simulink model "Test_simulation_model_backhoe"  (R2024a)
settings: Solver=FixedStepAuto  StartTime=0.0  StopTime=inf  FixedStep=0.0001  RelTol=1e-9
undefined symbols (not defined in the file or in its folder): X, Y, Z
libraries: sm_lib x67, nesl_utility x36, slpidlib x8
(part 3 of 4)

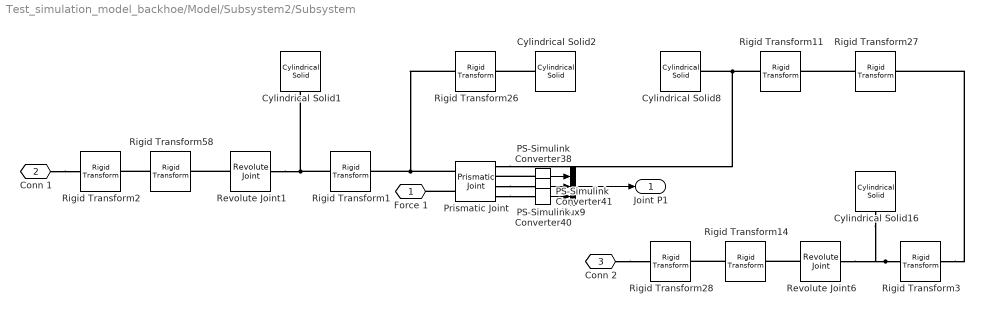
== system Test_simulation_model_backhoe/Model/Subsystem2/Subsystem ==
  Cylindrical Solid1 : sm_lib/Body Elements/Cylindrical Solid  CylinderRadius=0.05  CylinderRadiusUnits=m  CylinderLength=0.1  CylinderLengthUnits=m  ExportEntireGeometry=off  InertiaType=PointMass  BasedOnType=Density  Density=1000  DensityUnits=kg/m^3  Mass=0.0001  MassUnits=kg  CenterOfMass=[0 0 0]  CenterOfMassUnits=m  MomentsOfInertia=[1 1 1]  MomentsOfInertiaUnits=kg*m^2  ProductsOfInertia=[0 0 0]  ProductsOfInertiaUnits=kg*m^2  GraphicType=FromGeometry  MarkerShape=Sphere  MarkerSize=10  GraphicVisPropType=SimpleVisualProperties  GraphicDiffuseColor=[0.8 0.4 1.0]  GraphicOpacity=1.0  GraphicSpecularColor=[0.5 0.5 0.5 1.0]  GraphicAmbientColor=[0.15 0.15 0.15 1.0]  GraphicEmissiveColor=[0.0 0.0 0.0 1.0]  GraphicShininess=75  DoExposeReferenceFrame=on  SerializedFrames=<Frames/>
  Cylindrical Solid16 : sm_lib/Body Elements/Cylindrical Solid  CylinderRadius=0.05  CylinderRadiusUnits=m  CylinderLength=0.1  CylinderLengthUnits=m  ExportEntireGeometry=off  InertiaType=PointMass  BasedOnType=Density  Density=1000  DensityUnits=kg/m^3  Mass=0.00001  MassUnits=kg  CenterOfMass=[0 0 0]  CenterOfMassUnits=m  MomentsOfInertia=[1 1 1]  MomentsOfInertiaUnits=kg*m^2  ProductsOfInertia=[0 0 0]  ProductsOfInertiaUnits=kg*m^2  GraphicType=FromGeometry  MarkerShape=Sphere  MarkerSize=10  GraphicVisPropType=SimpleVisualProperties  GraphicDiffuseColor=[0.8 0.4 1.0]  GraphicOpacity=1.0  GraphicSpecularColor=[0.5 0.5 0.5 1.0]  GraphicAmbientColor=[0.15 0.15 0.15 1.0]  GraphicEmissiveColor=[0.0 0.0 0.0 1.0]  GraphicShininess=75  DoExposeReferenceFrame=on  SerializedFrames=<Frames/>
  Cylindrical Solid2 : sm_lib/Body Elements/Cylindrical Solid  CylinderRadius=0.02  CylinderRadiusUnits=m  CylinderLength=0.4  CylinderLengthUnits=m  ExportEntireGeometry=off  InertiaType=PointMass  BasedOnType=Density  Density=1000  DensityUnits=kg/m^3  Mass=0.001  MassUnits=kg  CenterOfMass=[0 0 0]  CenterOfMassUnits=m  MomentsOfInertia=[1 1 1]  MomentsOfInertiaUnits=kg*m^2  ProductsOfInertia=[0 0 0]  ProductsOfInertiaUnits=kg*m^2  GraphicType=FromGeometry  MarkerShape=Sphere  MarkerSize=10  GraphicVisPropType=SimpleVisualProperties  GraphicDiffuseColor=[0.0 0.8 0.6]  GraphicOpacity=1.0  GraphicSpecularColor=[0.5 0.5 0.5 1.0]  GraphicAmbientColor=[0.15 0.15 0.15 1.0]  GraphicEmissiveColor=[0.0 0.0 0.0 1.0]  GraphicShininess=75  DoExposeReferenceFrame=on  SerializedFrames=<Frames/>
  Cylindrical Solid8 : sm_lib/Body Elements/Cylindrical Solid  CylinderRadius=0.01  CylinderRadiusUnits=m  CylinderLength=0.55  CylinderLengthUnits=m  ExportEntireGeometry=off  InertiaType=PointMass  BasedOnType=Density  Density=1000  DensityUnits=kg/m^3  Mass=0.001  MassUnits=kg  CenterOfMass=[0 0 0]  CenterOfMassUnits=m  MomentsOfInertia=[1 1 1]  MomentsOfInertiaUnits=kg*m^2  ProductsOfInertia=[0 0 0]  ProductsOfInertiaUnits=kg*m^2  GraphicType=FromGeometry  MarkerShape=Sphere  MarkerSize=10  GraphicVisPropType=SimpleVisualProperties  GraphicDiffuseColor=[0.2 0.8 1.0]  GraphicOpacity=1.0  GraphicSpecularColor=[0.5 0.5 0.5 1.0]  GraphicAmbientColor=[0.15 0.15 0.15 1.0]  GraphicEmissiveColor=[0.0 0.0 0.0 1.0]  GraphicShininess=75  DoExposeReferenceFrame=on  SerializedFrames=<Frames/>
  Mux9 : Mux  Inputs=3
  PS-Simulink Converter38 : nesl_utility/PS-Simulink Converter  PhysicalDomain=network_engine_domain  SubClassName=ps_output  LeftPortType=input  RightPortType=output  PseudoPeriodic=off  Frequencies=[]  VectorFormat=inherit  Unit=inherit  AffineConversion=off
  PS-Simulink Converter40 : nesl_utility/PS-Simulink Converter  PhysicalDomain=network_engine_domain  SubClassName=ps_output  LeftPortType=input  RightPortType=output  PseudoPeriodic=off  Frequencies=[]  VectorFormat=inherit  Unit=inherit  AffineConversion=off
  PS-Simulink Converter41 : nesl_utility/PS-Simulink Converter  PhysicalDomain=network_engine_domain  SubClassName=ps_output  LeftPortType=input  RightPortType=output  PseudoPeriodic=off  Frequencies=[]  VectorFormat=inherit  Unit=inherit  AffineConversion=off
  Prismatic Joint : sm_lib/Joints/Prismatic Joint  JointMode=Normal  CompositeWrenchDir=FollowerOnBase  CompositeWrenchFrame=BaseFrame  SenseConstraintForce=off  SenseConstraintTorque=off  SenseTotalForce=off  SenseTotalTorque=off  PositionTargetSpecify=off  PositionTargetPriority=High  PositionTargetValue=0  PositionTargetValueUnits=m  VelocityTargetSpecify=off  VelocityTargetPriority=High  VelocityTargetValue=0  VelocityTargetValueUnits=m/s  EquilibriumPosition=0  EquilibriumPositionUnits=m  SpringStiffness=0  SpringStiffnessUnits=N/m  DampingCoefficient=0  DampingCoefficientUnits=N/(m/s)  LowerLimitSpecify=on  LowerLimitBound=0.25  LowerLimitBoundUnits=m  LowerLimitStiffness=1e6  LowerLimitStiffnessUnits=N/m  LowerLimitDamping=1e3  LowerLimitDampingUnits=N/(m/s)  LowerLimitTransitionRegionWidth=1e-4  LowerLimitTransitionRegionWidthUnits=m  UpperLimitSpecify=on  UpperLimitBound=0.6  UpperLimitBoundUnits=m  UpperLimitStiffness=1e6  UpperLimitStiffnessUnits=N/m  UpperLimitDamping=1e3  UpperLimitDampingUnits=N/(m/s)  UpperLimitTransitionRegionWidth=1e-4  UpperLimitTransitionRegionWidthUnits=m  TorqueActuationMode=InputTorque  MotionActuationMode=ComputedMotion  SensePosition=on  SenseVelocity=on  SenseAcceleration=off  SenseTorqueForce=on  SenseLowerLimitTorqueForce=off  SenseUpperLimitTorqueForce=off
  Revolute Joint1 : sm_lib/Joints/Revolute Joint  JointMode=Normal  CompositeWrenchDir=FollowerOnBase  CompositeWrenchFrame=BaseFrame  SenseConstraintForce=off  SenseConstraintTorque=off  SenseTotalForce=off  SenseTotalTorque=off  PositionTargetSpecify=on  PositionTargetPriority=Low  PositionTargetValue=-60  PositionTargetValueUnits=deg  VelocityTargetSpecify=off  VelocityTargetPriority=High  VelocityTargetValue=0  VelocityTargetValueUnits=deg/s  EquilibriumPosition=0  EquilibriumPositionUnits=deg  SpringStiffness=0  SpringStiffnessUnits=N*m/deg  DampingCoefficient=0  DampingCoefficientUnits=N*m/(deg/s)  LowerLimitSpecify=off  LowerLimitBound=-2  LowerLimitBoundUnits=deg  LowerLimitStiffness=1e4  LowerLimitStiffnessUnits=N*m/deg  LowerLimitDamping=10  LowerLimitDampingUnits=N*m/(deg/s)  LowerLimitTransitionRegionWidth=0.1  LowerLimitTransitionRegionWidthUnits=deg  UpperLimitSpecify=off  UpperLimitBound=-1  UpperLimitBoundUnits=deg  UpperLimitStiffness=1e4  UpperLimitStiffnessUnits=N*m/deg  UpperLimitDamping=10  UpperLimitDampingUnits=N*m/(deg/s)  UpperLimitTransitionRegionWidth=0.1  UpperLimitTransitionRegionWidthUnits=deg  TorqueActuationMode=NoTorque  MotionActuationMode=ComputedMotion  SensePosition=off  SenseVelocity=off  SenseAcceleration=off  SenseTorqueForce=off  SenseLowerLimitTorqueForce=off  SenseUpperLimitTorqueForce=off
  Revolute Joint6 : sm_lib/Joints/Revolute Joint  JointMode=Normal  CompositeWrenchDir=FollowerOnBase  CompositeWrenchFrame=BaseFrame  SenseConstraintForce=off  SenseConstraintTorque=off  SenseTotalForce=off  SenseTotalTorque=off  PositionTargetSpecify=off  PositionTargetPriority=High  PositionTargetValue=0  PositionTargetValueUnits=deg  VelocityTargetSpecify=off  VelocityTargetPriority=High  VelocityTargetValue=0  VelocityTargetValueUnits=deg/s  EquilibriumPosition=0  EquilibriumPositionUnits=deg  SpringStiffness=0  SpringStiffnessUnits=N*m/deg  DampingCoefficient=0  DampingCoefficientUnits=N*m/(deg/s)  LowerLimitSpecify=off  LowerLimitBound=-90  LowerLimitBoundUnits=deg  LowerLimitStiffness=1e4  LowerLimitStiffnessUnits=N*m/deg  LowerLimitDamping=10  LowerLimitDampingUnits=N*m/(deg/s)  LowerLimitTransitionRegionWidth=0.1  LowerLimitTransitionRegionWidthUnits=deg  UpperLimitSpecify=off  UpperLimitBound=90  UpperLimitBoundUnits=deg  UpperLimitStiffness=1e4  UpperLimitStiffnessUnits=N*m/deg  UpperLimitDamping=10  UpperLimitDampingUnits=N*m/(deg/s)  UpperLimitTransitionRegionWidth=0.1  UpperLimitTransitionRegionWidthUnits=deg  TorqueActuationMode=NoTorque  MotionActuationMode=ComputedMotion  SensePosition=off  SenseVelocity=off  SenseAcceleration=off  SenseTorqueForce=off  SenseLowerLimitTorqueForce=off  SenseUpperLimitTorqueForce=off
  Rigid Transform1 : sm_lib/Frames and Transforms/Rigid Transform  RotationMethod=StandardAxis  FollAlignAxisA=+X  BaseAlignAxisA=+Y  FollAlignAxisB=+Y  BaseAlignAxisB=+Z  RotationStandardAxis=-X  RotationAngle=90  RotationAngleUnits=deg  RotationArbitraryAxis=[0 0 1]  RotationSequenceAxes=FollowerAxes  RotationSequence=XYX  RotationSequenceAngles=[0 0 0]  RotationSequenceAnglesUnits=deg  RotationMatrix=[1 0 0; 0 1 0; 0 0 1]  Quaternion=[1 0 0 0]  TranslationMethod=Cartesian  TranslationCartesianOffset=[0 0 0]  TranslationCartesianOffsetUnits=m  TranslationStandardAxis=+Z  TranslationStandardOffset=0  TranslationStandardOffsetUnits=m  TranslationROffset=0  TranslationROffsetUnits=m  TranslationThetaOffset=0  TranslationThetaOffsetUnits=deg  TranslationZOffset=0  TranslationZOffsetUnits=m
  Rigid Transform11 : sm_lib/Frames and Transforms/Rigid Transform  RotationMethod=StandardAxis  FollAlignAxisA=+X  BaseAlignAxisA=+Y  FollAlignAxisB=+Y  BaseAlignAxisB=+Z  RotationStandardAxis=-Z  RotationAngle=90  RotationAngleUnits=deg  RotationArbitraryAxis=[0 0 1]  RotationSequenceAxes=FollowerAxes  RotationSequence=XYX  RotationSequenceAngles=[0 0 0]  RotationSequenceAnglesUnits=deg  RotationMatrix=[1 0 0; 0 1 0; 0 0 1]  Quaternion=[1 0 0 0]  TranslationMethod=Cartesian  TranslationCartesianOffset=[0 0 0]  TranslationCartesianOffsetUnits=m  TranslationStandardAxis=+Z  TranslationStandardOffset=0  TranslationStandardOffsetUnits=m  TranslationROffset=0  TranslationROffsetUnits=m  TranslationThetaOffset=0  TranslationThetaOffsetUnits=deg  TranslationZOffset=0  TranslationZOffsetUnits=m
  Rigid Transform14 : sm_lib/Frames and Transforms/Rigid Transform  RotationMethod=StandardAxis  FollAlignAxisA=+X  BaseAlignAxisA=+Y  FollAlignAxisB=+Y  BaseAlignAxisB=+Z  RotationStandardAxis=-Y  RotationAngle=90  RotationAngleUnits=deg  RotationArbitraryAxis=[0 0 1]  RotationSequenceAxes=FollowerAxes  RotationSequence=XYX  RotationSequenceAngles=[0 0 0]  RotationSequenceAnglesUnits=deg  RotationMatrix=[1 0 0; 0 1 0; 0 0 1]  Quaternion=[1 0 0 0]  TranslationMethod=Cartesian  TranslationCartesianOffset=[0 0 0]  TranslationCartesianOffsetUnits=m  TranslationStandardAxis=+Z  TranslationStandardOffset=0  TranslationStandardOffsetUnits=m  TranslationROffset=0  TranslationROffsetUnits=m  TranslationThetaOffset=0  TranslationThetaOffsetUnits=deg  TranslationZOffset=0  TranslationZOffsetUnits=m
  Rigid Transform2 : sm_lib/Frames and Transforms/Rigid Transform  RotationMethod=StandardAxis  FollAlignAxisA=+X  BaseAlignAxisA=+Y  FollAlignAxisB=+Y  BaseAlignAxisB=+Z  RotationStandardAxis=-Y  RotationAngle=90  RotationAngleUnits=deg  RotationArbitraryAxis=[0 0 1]  RotationSequenceAxes=FollowerAxes  RotationSequence=XYX  RotationSequenceAngles=[0 0 0]  RotationSequenceAnglesUnits=deg  RotationMatrix=[1 0 0; 0 1 0; 0 0 1]  Quaternion=[1 0 0 0]  TranslationMethod=Cartesian  TranslationCartesianOffset=[0 0 0]  TranslationCartesianOffsetUnits=m  TranslationStandardAxis=+Z  TranslationStandardOffset=0  TranslationStandardOffsetUnits=m  TranslationROffset=0  TranslationROffsetUnits=m  TranslationThetaOffset=0  TranslationThetaOffsetUnits=deg  TranslationZOffset=0  TranslationZOffsetUnits=m
  Rigid Transform26 : sm_lib/Frames and Transforms/Rigid Transform  RotationMethod=None  FollAlignAxisA=+X  BaseAlignAxisA=+Y  FollAlignAxisB=+Y  BaseAlignAxisB=+Z  RotationStandardAxis=+Y  RotationAngle=90  RotationAngleUnits=deg  RotationArbitraryAxis=[0 0 1]  RotationSequenceAxes=FollowerAxes  RotationSequence=XYX  RotationSequenceAngles=[0 0 0]  RotationSequenceAnglesUnits=deg  RotationMatrix=[1 0 0; 0 1 0; 0 0 1]  Quaternion=[1 0 0 0]  TranslationMethod=Cartesian  TranslationCartesianOffset=[0 0 0.2]  TranslationCartesianOffsetUnits=m  TranslationStandardAxis=+Z  TranslationStandardOffset=0  TranslationStandardOffsetUnits=m  TranslationROffset=0  TranslationROffsetUnits=m  TranslationThetaOffset=0  TranslationThetaOffsetUnits=deg  TranslationZOffset=0  TranslationZOffsetUnits=m
  Rigid Transform27 : sm_lib/Frames and Transforms/Rigid Transform  RotationMethod=None  FollAlignAxisA=+X  BaseAlignAxisA=+Y  FollAlignAxisB=+Y  BaseAlignAxisB=+Z  RotationStandardAxis=+Y  RotationAngle=90  RotationAngleUnits=deg  RotationArbitraryAxis=[0 0 1]  RotationSequenceAxes=FollowerAxes  RotationSequence=XYX  RotationSequenceAngles=[0 0 0]  RotationSequenceAnglesUnits=deg  RotationMatrix=[1 0 0; 0 1 0; 0 0 1]  Quaternion=[1 0 0 0]  TranslationMethod=Cartesian  TranslationCartesianOffset=[0 0 -0.3]  TranslationCartesianOffsetUnits=m  TranslationStandardAxis=+Z  TranslationStandardOffset=0  TranslationStandardOffsetUnits=m  TranslationROffset=0  TranslationROffsetUnits=m  TranslationThetaOffset=0  TranslationThetaOffsetUnits=deg  TranslationZOffset=0  TranslationZOffsetUnits=m
  Rigid Transform28 : sm_lib/Frames and Transforms/Rigid Transform  RotationMethod=None  FollAlignAxisA=+X  BaseAlignAxisA=+Y  FollAlignAxisB=+Y  BaseAlignAxisB=+Z  RotationStandardAxis=+Y  RotationAngle=90  RotationAngleUnits=deg  RotationArbitraryAxis=[0 0 1]  RotationSequenceAxes=FollowerAxes  RotationSequence=XYX  RotationSequenceAngles=[0 0 0]  RotationSequenceAnglesUnits=deg  RotationMatrix=[1 0 0; 0 1 0; 0 0 1]  Quaternion=[1 0 0 0]  TranslationMethod=Cartesian  TranslationCartesianOffset=[0 0 0.5]  TranslationCartesianOffsetUnits=m  TranslationStandardAxis=+Z  TranslationStandardOffset=0  TranslationStandardOffsetUnits=m  TranslationROffset=0  TranslationROffsetUnits=m  TranslationThetaOffset=0  TranslationThetaOffsetUnits=deg  TranslationZOffset=0  TranslationZOffsetUnits=m
  Rigid Transform3 : sm_lib/Frames and Transforms/Rigid Transform  RotationMethod=StandardAxis  FollAlignAxisA=+X  BaseAlignAxisA=+Y  FollAlignAxisB=+Y  BaseAlignAxisB=+Z  RotationStandardAxis=+Y  RotationAngle=90  RotationAngleUnits=deg  RotationArbitraryAxis=[0 0 1]  RotationSequenceAxes=FollowerAxes  RotationSequence=XYX  RotationSequenceAngles=[0 0 0]  RotationSequenceAnglesUnits=deg  RotationMatrix=[1 0 0; 0 1 0; 0 0 1]  Quaternion=[1 0 0 0]  TranslationMethod=Cartesian  TranslationCartesianOffset=[0 0 0]  TranslationCartesianOffsetUnits=m  TranslationStandardAxis=+Z  TranslationStandardOffset=0  TranslationStandardOffsetUnits=m  TranslationROffset=0  TranslationROffsetUnits=m  TranslationThetaOffset=0  TranslationThetaOffsetUnits=deg  TranslationZOffset=0  TranslationZOffsetUnits=m
  Rigid Transform58 : sm_lib/Frames and Transforms/Rigid Transform  RotationMethod=None  FollAlignAxisA=+X  BaseAlignAxisA=+Y  FollAlignAxisB=+Y  BaseAlignAxisB=+Z  RotationStandardAxis=-Y  RotationAngle=90  RotationAngleUnits=deg  RotationArbitraryAxis=[0 0 1]  RotationSequenceAxes=FollowerAxes  RotationSequence=XYX  RotationSequenceAngles=[0 0 0]  RotationSequenceAnglesUnits=deg  RotationMatrix=[1 0 0; 0 1 0; 0 0 1]  Quaternion=[1 0 0 0]  TranslationMethod=Cartesian  TranslationCartesianOffset=[0 0 0]  TranslationCartesianOffsetUnits=m  TranslationStandardAxis=+Z  TranslationStandardOffset=0  TranslationStandardOffsetUnits=m  TranslationROffset=0  TranslationROffsetUnits=m  TranslationThetaOffset=0  TranslationThetaOffsetUnits=deg  TranslationZOffset=0  TranslationZOffsetUnits=m
  Force 1 : PMIOPort  Side=Left
  Conn 1 : PMIOPort  Port=2  Side=Left
  Conn 2 : PMIOPort  Port=3  Side=Left
  Joint P1 : Outport
  wires:
  PS-Simulink Converter40/1 -> Mux9/2
  PS-Simulink Converter38/1 -> Mux9/1
  Mux9/1 -> Joint P1/1
  PS-Simulink Converter41/1 -> Mux9/3
  connections:
  Rigid Transform26/LConn1 -- Prismatic Joint/LConn1 -- Rigid Transform1/RConn1
  Rigid Transform27/RConn1 -- Rigid Transform11/LConn1
  PS-Simulink Converter38/LConn1 -- Prismatic Joint/RConn2
  Rigid Transform11/RConn1 -- Prismatic Joint/RConn1 -- Cylindrical Solid8/RConn1
  Rigid Transform58/LConn1 -- Rigid Transform2/RConn1
  Revolute Joint6/LConn1 -- Rigid Transform14/RConn1
  Rigid Transform3/RConn1 -- Rigid Transform27/LConn1
  Rigid Transform3/LConn1 -- Cylindrical Solid16/RConn1 -- Revolute Joint6/RConn1
  Cylindrical Solid2/RConn1 -- Rigid Transform26/RConn1
  Rigid Transform14/LConn1 -- Rigid Transform28/RConn1
  Conn 2/RConn1 -- Rigid Transform28/LConn1
  Rigid Transform1/LConn1 -- Revolute Joint1/RConn1 -- Cylindrical Solid1/RConn1
  Conn 1/RConn1 -- Rigid Transform2/LConn1
  Revolute Joint1/LConn1 -- Rigid Transform58/RConn1
  Prismatic Joint/RConn4 -- PS-Simulink Converter41/LConn1
  Prismatic Joint/RConn3 -- PS-Simulink Converter40/LConn1
  Prismatic Joint/LConn2 -- Force 1/RConn1

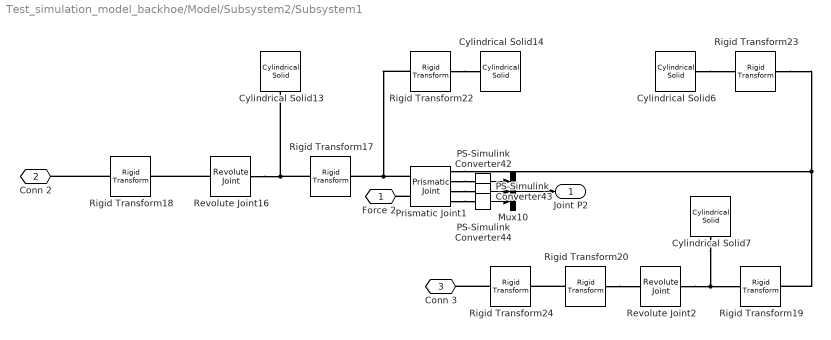
== system Test_simulation_model_backhoe/Model/Subsystem2/Subsystem1 ==
  Cylindrical Solid13 : sm_lib/Body Elements/Cylindrical Solid  CylinderRadius=0.05  CylinderRadiusUnits=m  CylinderLength=0.1  CylinderLengthUnits=m  ExportEntireGeometry=off  InertiaType=PointMass  BasedOnType=Density  Density=1000  DensityUnits=kg/m^3  Mass=0.00001  MassUnits=kg  CenterOfMass=[0 0 0]  CenterOfMassUnits=m  MomentsOfInertia=[1 1 1]  MomentsOfInertiaUnits=kg*m^2  ProductsOfInertia=[0 0 0]  ProductsOfInertiaUnits=kg*m^2  GraphicType=FromGeometry  MarkerShape=Sphere  MarkerSize=10  GraphicVisPropType=SimpleVisualProperties  GraphicDiffuseColor=[0.8 0.4 1.0]  GraphicOpacity=1.0  GraphicSpecularColor=[0.5 0.5 0.5 1.0]  GraphicAmbientColor=[0.15 0.15 0.15 1.0]  GraphicEmissiveColor=[0.0 0.0 0.0 1.0]  GraphicShininess=75  DoExposeReferenceFrame=on  SerializedFrames=<Frames/>
  Cylindrical Solid14 : sm_lib/Body Elements/Cylindrical Solid  CylinderRadius=0.02  CylinderRadiusUnits=m  CylinderLength=0.3  CylinderLengthUnits=m  ExportEntireGeometry=off  InertiaType=PointMass  BasedOnType=Density  Density=1000  DensityUnits=kg/m^3  Mass=0.001  MassUnits=kg  CenterOfMass=[0 0 0]  CenterOfMassUnits=m  MomentsOfInertia=[1 1 1]  MomentsOfInertiaUnits=kg*m^2  ProductsOfInertia=[0 0 0]  ProductsOfInertiaUnits=kg*m^2  GraphicType=FromGeometry  MarkerShape=Sphere  MarkerSize=10  GraphicVisPropType=SimpleVisualProperties  GraphicDiffuseColor=[0.0 0.8 0.6]  GraphicOpacity=1.0  GraphicSpecularColor=[0.5 0.5 0.5 1.0]  GraphicAmbientColor=[0.15 0.15 0.15 1.0]  GraphicEmissiveColor=[0.0 0.0 0.0 1.0]  GraphicShininess=75  DoExposeReferenceFrame=on  SerializedFrames=<Frames/>
  Cylindrical Solid6 : sm_lib/Body Elements/Cylindrical Solid  CylinderRadius=0.01  CylinderRadiusUnits=m  CylinderLength=0.5  CylinderLengthUnits=m  ExportEntireGeometry=off  InertiaType=PointMass  BasedOnType=Density  Density=1000  DensityUnits=kg/m^3  Mass=0.001  MassUnits=kg  CenterOfMass=[0 0 0]  CenterOfMassUnits=m  MomentsOfInertia=[1 1 1]  MomentsOfInertiaUnits=kg*m^2  ProductsOfInertia=[0 0 0]  ProductsOfInertiaUnits=kg*m^2  GraphicType=FromGeometry  MarkerShape=Sphere  MarkerSize=10  GraphicVisPropType=SimpleVisualProperties  GraphicDiffuseColor=[0.2 0.8 1.0]  GraphicOpacity=1.0  GraphicSpecularColor=[0.5 0.5 0.5 1.0]  GraphicAmbientColor=[0.15 0.15 0.15 1.0]  GraphicEmissiveColor=[0.0 0.0 0.0 1.0]  GraphicShininess=75  DoExposeReferenceFrame=on  SerializedFrames=<Frames/>
  Cylindrical Solid7 : sm_lib/Body Elements/Cylindrical Solid  CylinderRadius=0.05  CylinderRadiusUnits=m  CylinderLength=0.1  CylinderLengthUnits=m  ExportEntireGeometry=off  InertiaType=PointMass  BasedOnType=Density  Density=1000  DensityUnits=kg/m^3  Mass=0.00001  MassUnits=kg  CenterOfMass=[0 0 0]  CenterOfMassUnits=m  MomentsOfInertia=[1 1 1]  MomentsOfInertiaUnits=kg*m^2  ProductsOfInertia=[0 0 0]  ProductsOfInertiaUnits=kg*m^2  GraphicType=FromGeometry  MarkerShape=Sphere  MarkerSize=10  GraphicVisPropType=SimpleVisualProperties  GraphicDiffuseColor=[0.8 0.4 1.0]  GraphicOpacity=1.0  GraphicSpecularColor=[0.5 0.5 0.5 1.0]  GraphicAmbientColor=[0.15 0.15 0.15 1.0]  GraphicEmissiveColor=[0.0 0.0 0.0 1.0]  GraphicShininess=75  DoExposeReferenceFrame=on  SerializedFrames=<Frames/>
  Mux10 : Mux  Inputs=3
  PS-Simulink Converter42 : nesl_utility/PS-Simulink Converter  PhysicalDomain=network_engine_domain  SubClassName=ps_output  LeftPortType=input  RightPortType=output  PseudoPeriodic=off  Frequencies=[]  VectorFormat=inherit  Unit=inherit  AffineConversion=off
  PS-Simulink Converter43 : nesl_utility/PS-Simulink Converter  PhysicalDomain=network_engine_domain  SubClassName=ps_output  LeftPortType=input  RightPortType=output  PseudoPeriodic=off  Frequencies=[]  VectorFormat=inherit  Unit=inherit  AffineConversion=off
  PS-Simulink Converter44 : nesl_utility/PS-Simulink Converter  PhysicalDomain=network_engine_domain  SubClassName=ps_output  LeftPortType=input  RightPortType=output  PseudoPeriodic=off  Frequencies=[]  VectorFormat=inherit  Unit=inherit  AffineConversion=off
  Prismatic Joint1 : sm_lib/Joints/Prismatic Joint  JointMode=Normal  CompositeWrenchDir=FollowerOnBase  CompositeWrenchFrame=BaseFrame  SenseConstraintForce=off  SenseConstraintTorque=off  SenseTotalForce=off  SenseTotalTorque=off  PositionTargetSpecify=off  PositionTargetPriority=High  PositionTargetValue=0  PositionTargetValueUnits=m  VelocityTargetSpecify=off  VelocityTargetPriority=High  VelocityTargetValue=0  VelocityTargetValueUnits=m/s  EquilibriumPosition=0  EquilibriumPositionUnits=m  SpringStiffness=0  SpringStiffnessUnits=N/m  DampingCoefficient=0  DampingCoefficientUnits=N/(m/s)  LowerLimitSpecify=on  LowerLimitBound=-0.8  LowerLimitBoundUnits=m  LowerLimitStiffness=1e6  LowerLimitStiffnessUnits=N/m  LowerLimitDamping=1e3  LowerLimitDampingUnits=N/(m/s)  LowerLimitTransitionRegionWidth=1e-4  LowerLimitTransitionRegionWidthUnits=m  UpperLimitSpecify=on  UpperLimitBound=-0.4  UpperLimitBoundUnits=m  UpperLimitStiffness=1e6  UpperLimitStiffnessUnits=N/m  UpperLimitDamping=1e3  UpperLimitDampingUnits=N/(m/s)  UpperLimitTransitionRegionWidth=1e-4  UpperLimitTransitionRegionWidthUnits=m  TorqueActuationMode=InputTorque  MotionActuationMode=ComputedMotion  SensePosition=on  SenseVelocity=on  SenseAcceleration=off  SenseTorqueForce=on  SenseLowerLimitTorqueForce=off  SenseUpperLimitTorqueForce=off
  Revolute Joint16 : sm_lib/Joints/Revolute Joint  JointMode=Normal  CompositeWrenchDir=FollowerOnBase  CompositeWrenchFrame=BaseFrame  SenseConstraintForce=off  SenseConstraintTorque=off  SenseTotalForce=off  SenseTotalTorque=off  PositionTargetSpecify=on  PositionTargetPriority=High  PositionTargetValue=10  PositionTargetValueUnits=deg  VelocityTargetSpecify=off  VelocityTargetPriority=High  VelocityTargetValue=0  VelocityTargetValueUnits=deg/s  EquilibriumPosition=0  EquilibriumPositionUnits=deg  SpringStiffness=0  SpringStiffnessUnits=N*m/deg  DampingCoefficient=0  DampingCoefficientUnits=N*m/(deg/s)  LowerLimitSpecify=off  LowerLimitBound=-45  LowerLimitBoundUnits=deg  LowerLimitStiffness=1e4  LowerLimitStiffnessUnits=N*m/deg  LowerLimitDamping=10  LowerLimitDampingUnits=N*m/(deg/s)  LowerLimitTransitionRegionWidth=0.1  LowerLimitTransitionRegionWidthUnits=deg  UpperLimitSpecify=off  UpperLimitBound=60  UpperLimitBoundUnits=deg  UpperLimitStiffness=1e4  UpperLimitStiffnessUnits=N*m/deg  UpperLimitDamping=10  UpperLimitDampingUnits=N*m/(deg/s)  UpperLimitTransitionRegionWidth=0.1  UpperLimitTransitionRegionWidthUnits=deg  TorqueActuationMode=NoTorque  MotionActuationMode=ComputedMotion  SensePosition=off  SenseVelocity=off  SenseAcceleration=off  SenseTorqueForce=off  SenseLowerLimitTorqueForce=off  SenseUpperLimitTorqueForce=off
  Revolute Joint2 : sm_lib/Joints/Revolute Joint  JointMode=Normal  CompositeWrenchDir=FollowerOnBase  CompositeWrenchFrame=BaseFrame  SenseConstraintForce=off  SenseConstraintTorque=off  SenseTotalForce=off  SenseTotalTorque=off  PositionTargetSpecify=off  PositionTargetPriority=High  PositionTargetValue=0  PositionTargetValueUnits=deg  VelocityTargetSpecify=off  VelocityTargetPriority=High  VelocityTargetValue=0  VelocityTargetValueUnits=deg/s  EquilibriumPosition=0  EquilibriumPositionUnits=deg  SpringStiffness=0  SpringStiffnessUnits=N*m/deg  DampingCoefficient=0  DampingCoefficientUnits=N*m/(deg/s)  LowerLimitSpecify=off  LowerLimitBound=-90  LowerLimitBoundUnits=deg  LowerLimitStiffness=1e4  LowerLimitStiffnessUnits=N*m/deg  LowerLimitDamping=10  LowerLimitDampingUnits=N*m/(deg/s)  LowerLimitTransitionRegionWidth=0.1  LowerLimitTransitionRegionWidthUnits=deg  UpperLimitSpecify=off  UpperLimitBound=90  UpperLimitBoundUnits=deg  UpperLimitStiffness=1e4  UpperLimitStiffnessUnits=N*m/deg  UpperLimitDamping=10  UpperLimitDampingUnits=N*m/(deg/s)  UpperLimitTransitionRegionWidth=0.1  UpperLimitTransitionRegionWidthUnits=deg  TorqueActuationMode=NoTorque  MotionActuationMode=ComputedMotion  SensePosition=off  SenseVelocity=off  SenseAcceleration=off  SenseTorqueForce=off  SenseLowerLimitTorqueForce=off  SenseUpperLimitTorqueForce=off
  Rigid Transform17 : sm_lib/Frames and Transforms/Rigid Transform  RotationMethod=StandardAxis  FollAlignAxisA=+X  BaseAlignAxisA=+Y  FollAlignAxisB=+Y  BaseAlignAxisB=+Z  RotationStandardAxis=-X  RotationAngle=90  RotationAngleUnits=deg  RotationArbitraryAxis=[0 0 1]  RotationSequenceAxes=FollowerAxes  RotationSequence=XYX  RotationSequenceAngles=[0 0 0]  RotationSequenceAnglesUnits=deg  RotationMatrix=[1 0 0; 0 1 0; 0 0 1]  Quaternion=[1 0 0 0]  TranslationMethod=Cartesian  TranslationCartesianOffset=[0 0 0]  TranslationCartesianOffsetUnits=m  TranslationStandardAxis=+Z  TranslationStandardOffset=0  TranslationStandardOffsetUnits=m  TranslationROffset=0  TranslationROffsetUnits=m  TranslationThetaOffset=0  TranslationThetaOffsetUnits=deg  TranslationZOffset=0  TranslationZOffsetUnits=m
  Rigid Transform18 : sm_lib/Frames and Transforms/Rigid Transform  RotationMethod=StandardAxis  FollAlignAxisA=+X  BaseAlignAxisA=+Y  FollAlignAxisB=+Y  BaseAlignAxisB=+Z  RotationStandardAxis=-Y  RotationAngle=90  RotationAngleUnits=deg  RotationArbitraryAxis=[0 0 1]  RotationSequenceAxes=FollowerAxes  RotationSequence=XYX  RotationSequenceAngles=[0 0 0]  RotationSequenceAnglesUnits=deg  RotationMatrix=[1 0 0; 0 1 0; 0 0 1]  Quaternion=[1 0 0 0]  TranslationMethod=Cartesian  TranslationCartesianOffset=[0 0 0.85]  TranslationCartesianOffsetUnits=m  TranslationStandardAxis=+Z  TranslationStandardOffset=0  TranslationStandardOffsetUnits=m  TranslationROffset=0  TranslationROffsetUnits=m  TranslationThetaOffset=0  TranslationThetaOffsetUnits=deg  TranslationZOffset=0  TranslationZOffsetUnits=m
  Rigid Transform19 : sm_lib/Frames and Transforms/Rigid Transform  RotationMethod=StandardAxis  FollAlignAxisA=+X  BaseAlignAxisA=+Y  FollAlignAxisB=+Y  BaseAlignAxisB=+Z  RotationStandardAxis=+X  RotationAngle=90  RotationAngleUnits=deg  RotationArbitraryAxis=[0 0 1]  RotationSequenceAxes=FollowerAxes  RotationSequence=XYX  RotationSequenceAngles=[0 0 0]  RotationSequenceAnglesUnits=deg  RotationMatrix=[1 0 0; 0 1 0; 0 0 1]  Quaternion=[1 0 0 0]  TranslationMethod=Cartesian  TranslationCartesianOffset=[0 0 0]  TranslationCartesianOffsetUnits=m  TranslationStandardAxis=+Z  TranslationStandardOffset=0  TranslationStandardOffsetUnits=m  TranslationROffset=0  TranslationROffsetUnits=m  TranslationThetaOffset=0  TranslationThetaOffsetUnits=deg  TranslationZOffset=0  TranslationZOffsetUnits=m
  Rigid Transform20 : sm_lib/Frames and Transforms/Rigid Transform  RotationMethod=None  FollAlignAxisA=+X  BaseAlignAxisA=+Y  FollAlignAxisB=+Y  BaseAlignAxisB=+Z  RotationStandardAxis=-Y  RotationAngle=90  RotationAngleUnits=deg  RotationArbitraryAxis=[0 0 1]  RotationSequenceAxes=FollowerAxes  RotationSequence=XYX  RotationSequenceAngles=[0 0 0]  RotationSequenceAnglesUnits=deg  RotationMatrix=[1 0 0; 0 1 0; 0 0 1]  Quaternion=[1 0 0 0]  TranslationMethod=Cartesian  TranslationCartesianOffset=[0.125 0 0]  TranslationCartesianOffsetUnits=m  TranslationStandardAxis=+Z  TranslationStandardOffset=0  TranslationStandardOffsetUnits=m  TranslationROffset=0  TranslationROffsetUnits=m  TranslationThetaOffset=0  TranslationThetaOffsetUnits=deg  TranslationZOffset=0  TranslationZOffsetUnits=m
  Rigid Transform22 : sm_lib/Frames and Transforms/Rigid Transform  RotationMethod=None  FollAlignAxisA=+X  BaseAlignAxisA=+Y  FollAlignAxisB=+Y  BaseAlignAxisB=+Z  RotationStandardAxis=+Y  RotationAngle=90  RotationAngleUnits=deg  RotationArbitraryAxis=[0 0 1]  RotationSequenceAxes=FollowerAxes  RotationSequence=XYX  RotationSequenceAngles=[0 0 0]  RotationSequenceAnglesUnits=deg  RotationMatrix=[1 0 0; 0 1 0; 0 0 1]  Quaternion=[1 0 0 0]  TranslationMethod=Cartesian  TranslationCartesianOffset=[0 0 -0.2]  TranslationCartesianOffsetUnits=m  TranslationStandardAxis=+Z  TranslationStandardOffset=0  TranslationStandardOffsetUnits=m  TranslationROffset=0  TranslationROffsetUnits=m  TranslationThetaOffset=0  TranslationThetaOffsetUnits=deg  TranslationZOffset=0  TranslationZOffsetUnits=m
  Rigid Transform23 : sm_lib/Frames and Transforms/Rigid Transform  RotationMethod=None  FollAlignAxisA=+X  BaseAlignAxisA=+Y  FollAlignAxisB=+Y  BaseAlignAxisB=+Z  RotationStandardAxis=+Y  RotationAngle=90  RotationAngleUnits=deg  RotationArbitraryAxis=[0 0 1]  RotationSequenceAxes=FollowerAxes  RotationSequence=XYX  RotationSequenceAngles=[0 0 0]  RotationSequenceAnglesUnits=deg  RotationMatrix=[1 0 0; 0 1 0; 0 0 1]  Quaternion=[1 0 0 0]  TranslationMethod=Cartesian  TranslationCartesianOffset=[0 0 0.225]  TranslationCartesianOffsetUnits=m  TranslationStandardAxis=+Z  TranslationStandardOffset=0  TranslationStandardOffsetUnits=m  TranslationROffset=0  TranslationROffsetUnits=m  TranslationThetaOffset=0  TranslationThetaOffsetUnits=deg  TranslationZOffset=0  TranslationZOffsetUnits=m
  Rigid Transform24 : sm_lib/Frames and Transforms/Rigid Transform  RotationMethod=StandardAxis  FollAlignAxisA=+X  BaseAlignAxisA=+Y  FollAlignAxisB=+Y  BaseAlignAxisB=+Z  RotationStandardAxis=+Y  RotationAngle=90  RotationAngleUnits=deg  RotationArbitraryAxis=[0 0 1]  RotationSequenceAxes=FollowerAxes  RotationSequence=XYX  RotationSequenceAngles=[0 0 0]  RotationSequenceAnglesUnits=deg  RotationMatrix=[1 0 0; 0 1 0; 0 0 1]  Quaternion=[1 0 0 0]  TranslationMethod=Cartesian  TranslationCartesianOffset=[0 0 0]  TranslationCartesianOffsetUnits=m  TranslationStandardAxis=+Z  TranslationStandardOffset=0  TranslationStandardOffsetUnits=m  TranslationROffset=0  TranslationROffsetUnits=m  TranslationThetaOffset=0  TranslationThetaOffsetUnits=deg  TranslationZOffset=0  TranslationZOffsetUnits=m
  Force 2 : PMIOPort  Side=Left
  Conn 2 : PMIOPort  Port=2  Side=Left
  Conn 3 : PMIOPort  Port=3  Side=Left
  Joint P2 : Outport
  wires:
  PS-Simulink Converter44/1 -> Mux10/3
  PS-Simulink Converter43/1 -> Mux10/2
  PS-Simulink Converter42/1 -> Mux10/1
  Mux10/1 -> Joint P2/1
  connections:
  Cylindrical Solid7/RConn1 -- Revolute Joint2/RConn1 -- Rigid Transform19/LConn1
  Prismatic Joint1/RConn1 -- Rigid Transform19/RConn1 -- Rigid Transform23/LConn1
  Rigid Transform22/RConn1 -- Cylindrical Solid14/RConn1
  Cylindrical Solid6/RConn1 -- Rigid Transform23/RConn1
  Rigid Transform22/LConn1 -- Prismatic Joint1/LConn1 -- Rigid Transform17/RConn1
  Rigid Transform17/LConn1 -- Revolute Joint16/RConn1 -- Cylindrical Solid13/RConn1
  Prismatic Joint1/LConn2 -- Force 2/RConn1
  Prismatic Joint1/RConn3 -- PS-Simulink Converter43/LConn1
  Prismatic Joint1/RConn4 -- PS-Simulink Converter44/LConn1
  Prismatic Joint1/RConn2 -- PS-Simulink Converter42/LConn1
  Rigid Transform20/RConn1 -- Revolute Joint2/LConn1
  Revolute Joint16/LConn1 -- Rigid Transform18/RConn1
  Rigid Transform20/LConn1 -- Rigid Transform24/RConn1
  Rigid Transform18/LConn1 -- Conn 2/RConn1
  Rigid Transform24/LConn1 -- Conn 3/RConn1

== matlab function Test_simulation_model_backhoe/Dynamics1 ==
  data: q input; tau output; qd input; qdd input; m input; I1 input; I2 input; I3 input; I4 input
function tau = dynamics_4DOF(q, qd, qdd, m, I1, I2, I3, I4)
    % dynamics_4DOF: Calculates joint torques for a 4-DOF manipulator
    % Input:
    %   q: Joint angles [q1; q2; q3; q4]
    %   qd: Joint velocities [qd1; qd2; qd3; qd4]
    %   qdd: Joint accelerations [qdd1; qdd2; qdd3; qdd4]
    %   params: Struct with manipulator parameters
    %       params.m: Mass of links [m1, m2, m3, m4]
    %       params.L: Lengths of links [L1, L2, L3, L4]
    %       params.I: Inertia matrices for links (cell array of 3x3 matrices)
    %       params.g: Gravity (e.g., 9.81 m/s^2)
    % Output:
    %   tau: Joint torques [tau1; tau2; tau3; tau4]

    % กำหนดขนาดของเอาต์พุต
    tau = zeros(4, 1); % กำหนดให้ tau เป็นเวกเตอร์ขนาด 4x1

    assert(isequal(size(q), [4, 1]));      % กำหนดว่า q ต้องมีขนาด 4x1
    assert(isequal(size(qd), [4, 1]));     % qd ต้องมีขนาด 4x1
    assert(isequal(size(qdd), [4, 1]));    % qdd ต้องมีขนาด 4x1
    assert(isequal(size(I1), [3, 3])); % inertiaMatrix ต้องเป็น 3x3
    assert(isequal(size(I2), [3, 3])); % inertiaMatrix ต้องเป็น 3x3
    assert(isequal(size(I3), [3, 3])); % inertiaMatrix ต้องเป็น 3x3
    assert(isequal(size(I4), [3, 3])); % inertiaMatrix ต้องเป็น 3x3

    % Unpack parameters
    % m = params.m;    % Masses
    L = [0.25, 1, 1.5, 0.75];    % Link lengths
    I = [I1, I2, I3, I4];    % Cell array of inertia matrices (3x3)
    g = 9.81;    % Gravity acceleration

    % Joint variables
    q1 = q(1); q2 = q(2); q3 = q(3); q4 = q(4);
    qd1 = qd(1); qd2 = qd(2); qd3 = qd(3); qd4 = qd(4);
    qdd1 = qdd(1); qdd2 = qdd(2); qdd3 = qdd(3); qdd4 = qdd(4);

    % Gravitational forces
    G1 = m(1) * g * L(1) / 2 * cos(q1);
    G2 = m(2) * g * (L(1) * cos(q1) + L(2) / 2 * cos(q1 + q2));
    G3 = m(3) * g * (L(1) * cos(q1) + L(2) * cos(q1 + q2) + L(3) / 2 * cos(q1 + q2 + q3));
    G4 = m(4) * g * (L(1) * cos(q1) + L(2) * cos(q1 + q2) + L(3) * cos(q1 + q2 + q3) + L(4) / 2 * cos(q1 + q2 + q3 + q4));
    G = [G1; G2; G3; G4];

    % Inertia matrix
    M = zeros(4, 4);
    for i = 1:4
        M(i, i) = I(3, 3); % Use principal moment of inertia along z-axis
    end

    % Coriolis and Centrifugal forces (simplified)
    C = zeros(4, 4);

    % Compute torques
    tau = M * qdd + C * qd + G;
end

== matlab function Test_simulation_model_backhoe/Forward Kinematic ==
  data: joint_angles input; x output; y output; z output
function [x, y, z] = FK(joint_angles)
    % FK_Simulink: Calculates the position and orientation of the end effector for a 4-DOF manipulator

    % Lengths of the links
    d1 = 0.3;  % {0} -> {1}
    a1 = 0.2;  % {1} -> {2}
    L1 = 0.25; % Link 1
    L2 = 1;    % Link 2
    L3 = 1.5;  % Link 3
    L4 = 0.75; % Link 4 (End Effector)

    % Extract joint angles
    q1 = joint_angles(1); % Joint 1 (base rotation)
    q2 = joint_angles(2); % Joint 2 (shoulder rotation)
    q3 = joint_angles(3); % Joint 3 (elbow rotation)
    q4 = joint_angles(4); % Joint 4 (end effector orientation)

    x12 = pi/2;
    z23 = pi/2;

    % Transformation Matrices
    % Transform from base frame to end effector
    % Transformation for Joint 0 -> 1 (Rotation around the base)
    T01_T1 = [  1, 0, 0,  0;
                0, 1, 0,  0;
                0, 0, 1, d1;
                0, 0, 0,  1];

    T01_Rz = [  cos(q1), -sin(q1), 0, 0;
                sin(q1),  cos(q1), 0, 0;
                      0,        0, 1, 0;
                      0,        0, 0, 1];

    T01 = T01_T1 * T01_Rz;

    % Transformation for Joint 1 -> 2 (shoulder)
    T12_T1 = [  1, 0, 0, -a1;
                0, 1, 0,   0;
                0, 0, 1,  L1;
                0, 0, 0,   1];

    T12_Rx = [  1,        0,         0, 0;
                0, cos(x12), -sin(x12), 0;
                0, sin(x12),  cos(x12), 0;
                0,        0,         0, 1];

    T12_Rz = [  cos(q2), -sin(q2), 0, 0;
                sin(q2),  cos(q2), 0, 0;
                      0,        0, 1, 0;
                      0,        0, 0, 1];

    T12 = T12_T1 * T12_Rx * T12_Rz;

    % Transformation for Joint 2 -> 3 (elbow)
    T23_Rz1 = [  cos(z23), -sin(z23), 0, 0;
                 sin(z23),  cos(z23), 0, 0;
                        0,         0, 1, 0;
                        0,         0, 0, 1];

    T23_T1 = [  1, 0, 0, L2;
                0, 1, 0,  0;
                0, 0, 1,  0;
                0, 0, 0,  1];

    T23_Rz = [  cos(q3), -sin(q3), 0, 0;
                sin(q3),  cos(q3), 0, 0;
                      0,        0, 1, 0;
                      0,        0, 0, 1];

    T23 = T23_Rz1 * T23_T1 * T23_Rz;

    % Transformation for Joint 3 -> 4
    T34_T1 = [  1, 0, 0, L3;
                0, 1, 0,  0;
                0, 0, 1,  0;
                0, 0, 0,  1];

    T34_Rz = [  cos(q4), -sin(q4), 0, 0;
                sin(q4),  cos(q4), 0, 0;
                      0,        0, 1, 0;
                      0,        0, 0, 1];

    T34 = T34_T1 * T34_Rz;

    % Transformation for Joint 4 -> e

    T4e = [ 1, 0, 0, L4;
            0, 1, 0,  0;
            0, 0, 1,  0;
            0, 0, 0,  1];

    % Final transformation from the base to end effector
    T = T01 * T12 * T23 * T34 * T4e;

    % Extract position from the final transformation matrix
    x = T(1, 4); % x-position of the end effector
    y = T(2, 4); % y-position of the end effector
    z = T(3, 4); % z-position of the end effector

  
end

% Tranformation matrix
% ([  [-sin(q2 + q3 + q4)*cos(q1), -cos(q1)*cos(q2 + q3 + q4),  sin(q1), -L2*sin(q2)*cos(q1) - L3*sin(q2 + q3)*cos(q1) - L4*sin(q2 + q3 + q4)*cos(q1) - a1*cos(q1)], ...
%     [-sin(q1)*sin(q2 + q3 + q4), -sin(q1)*cos(q2 + q3 + q4), -cos(q1), -L2*sin(q1)*sin(q2) - L3*sin(q1)*sin(q2 + q3) - L4*sin(q1)*sin(q2 + q3 + q4) - a1*sin(q1)], ...
%     [         cos(q2 + q3 + q4),         -sin(q2 + q3 + q4),        0,                     L1 + L2*cos(q2) + L3*(1.0*cos(q2 + q3)) + L4*(cos(q2 + q3 + q4)) + d1], ...
%     [                         0,                          0,        0,                                                                                         1]  ])

== matlab function Test_simulation_model_backhoe/Trajectory/MATLAB Function ==
  data: qf input; q output; t input; qd output; qdd output
function [q, qd, qdd] = quintic_trajectory_planning(qf, t)
    % Quintic Trajectory Planning with reference to Simulink Clock for 3-second duration
    
    % Initial conditions (set to zero)
    q0 = 0;      % Initial Position
    qd0 = 0;     % Initial Velocity
    qdd0 = 0;    % Initial Acceleration
    qdf = 0;     % Final Velocity
    qddf = 0;    % Final Acceleration
    
    % Total time for trajectory
    T = 0.5;  % 3 seconds duration
    
    % Clamp time to ensure it does not exceed 3 seconds
    t = min(t, T);
    
    % Polynomial coefficients calculation based on boundary conditions
    a0 = q0;
    a1 = qd0;
    a2 = qdd0 / 2;
    a3 = (20 * qf - 20 * q0 - 8 * qdf - 12 * qd0 - 3 * qdd0 + qddf) / (2 * T^3);
    a4 = (30 * q0 - 30 * qf + 14 * qdf + 16 * qd0 + 3 * qdd0 - 2 * qddf) / (2 * T^4);
    a5 = (12 * qf - 12 * q0 - 6 * qdf - 6 * qd0 - qdd0 + qddf) / (2 * T^5);
    
    % Calculate position, velocity, and acceleration based on time t
    q = a0 + a1 * t + a2 * t^2 + a3 * t^3 + a4 * t^4 + a5 * t^5;
    qd = a1 + 2 * a2 * t + 3 * a3 * t^2 + 4 * a4 * t^3 + 5 * a5 * t^4;
    qdd = 2 * a2 + 6 * a3 * t + 12 * a4 * t^2 + 20 * a5 * t^3;
    
    % Ensure the final position q reaches qf exactly after 3 seconds
    if t == T
        q = qf;
        qd = 0;  % Final velocity is zero if not specified
        qdd = 0; % Final acceleration is zero if not specified
    end
end

== matlab function Test_simulation_model_backhoe/Trajectory/MATLAB Function1 ==
  data: qf input; q output; t input; qd output; qdd output
function [q, qd, qdd] = quintic_trajectory_planning(qf, t)
    % Quintic Trajectory Planning with reference to Simulink Clock for 3-second duration
    
    % Initial conditions (set to zero)
    q0 = 0;      % Initial Position
    qd0 = 0;     % Initial Velocity
    qdd0 = 0;    % Initial Acceleration
    qdf = 0;     % Final Velocity
    qddf = 0;    % Final Acceleration
    
    % Total time for trajectory
    T = 0.5;  % 3 seconds duration
    
    % Clamp time to ensure it does not exceed 3 seconds
    t = min(t, T);
    
    % Polynomial coefficients calculation based on boundary conditions
    a0 = q0;
    a1 = qd0;
    a2 = qdd0 / 2;
    a3 = (20 * qf - 20 * q0 - 8 * qdf - 12 * qd0 - 3 * qdd0 + qddf) / (2 * T^3);
    a4 = (30 * q0 - 30 * qf + 14 * qdf + 16 * qd0 + 3 * qdd0 - 2 * qddf) / (2 * T^4);
    a5 = (12 * qf - 12 * q0 - 6 * qdf - 6 * qd0 - qdd0 + qddf) / (2 * T^5);
    
    % Calculate position, velocity, and acceleration based on time t
    q = a0 + a1 * t + a2 * t^2 + a3 * t^3 + a4 * t^4 + a5 * t^5;
    qd = a1 + 2 * a2 * t + 3 * a3 * t^2 + 4 * a4 * t^3 + 5 * a5 * t^4;
    qdd = 2 * a2 + 6 * a3 * t + 12 * a4 * t^2 + 20 * a5 * t^3;
    
    % Ensure the final position q reaches qf exactly after 3 seconds
    if t == T
        q = qf;
        qd = 0;  % Final velocity is zero if not specified
        qdd = 0; % Final acceleration is zero if not specified
    end
end

== matlab function Test_simulation_model_backhoe/Inverse Kinematic ==
  data: x input; joint_angles output; y input; z input
function joint_angles = IK_Simulink(x, y, z)
    % Lengths of the links
    L1 = 0.25; % Link 1
    L2 = 1; % Link 2
    L3 = 1.5; % Link 3
    L4 = 0.75; % Link 4 (End Effector)
    d1 = 0.3;
    a1 = -0.2;

    x_target = x;
    y_target = y;
    z_target = z;

    q1 = atan2(y_target, x_target);
    sinq1 = sin(q1);
    cosq1 = cos(q1);

    A = x_target * cosq1 + y_target * sinq1 - a1 - L4;
    B = z_target - (d1 + L1) - L4;

    cosq3 = (A^2 + B^2 - L2^2 - L3^2) / (2 * L2 * L3);
    cosq3 = max(-1, min(1, cosq3));
    sinq3 = sqrt(1 - cosq3^2);

    C = L2 + L3 * cosq3;
    D = L3 * sinq3;

    sinq2 = (B * C - A * D) / (C^2 + D^2);
    cosq2 = sqrt(1 - sinq2^2);
    q2 = atan2(sinq2, cosq2);

    q3 = atan2(sinq3, cosq3);

    nz = cos(q2 + q3);
    oz = -sin(q2 + q3);
    q4 = atan2(nz, oz) - q2 - q3;

    joint_angles = [q1; q2; q3; q4];
end
% function joint_angles = IK(x, y, z)
%     % กำหนดขนาดคงที่สำหรับ output solutions
%     joint_angles = zeros(1, 4); % solutions จะมีขนาด [1x4] เสมอ
% 
%     % Lengths of the links
%     d1 = 0.3;  
%     a1 = 0.2;  
%     L1 = 0.25; 
%     L2 = 1;    
%     L3 = 1.5;  
%     L4 = 0.75; 
% 
%     % Initial guess for q1, q2, q3, q4
%     initial_guess = [0, 0, 0, 0];
% 
%     % Define the function to solve
%     function F = equations(vars)
%         q1 = vars(1);
%         q2 = vars(2);
%         q3 = vars(3);
%         q4 = vars(4);
%         F = [
%             -L2*sin(q2)*cos(q1) - L3*sin(q2 + q3)*cos(q1) - L4*sin(q2 + q3 + q4)*cos(q1) - a1*cos(q1) - x;
%             -L2*sin(q1)*sin(q2) - L3*sin(q1)*sin(q2 + q3) - L4*sin(q1)*sin(q2 + q3 + q4) - a1*sin(q1) - y;
%             L1 + L2*cos(q2) + L3*cos(q2 + q3) + L4*cos(q2 + q3 + q4) + d1 - z;
%         ];
%     end
% 
%     % Solve the equations numerically
%     options = optimoptions('fsolve', 'Algorithm', 'levenberg-marquardt', 'Display', 'none');
%     joint_angles = fsolve(@equations, initial_guess, options);
% end

== matlab function Test_simulation_model_backhoe/Trajectory/MATLAB Function2 ==
  data: qf input; q output; t input; qd output; qdd output
function [q, qd, qdd] = quintic_trajectory_planning(qf, t)
    % Quintic Trajectory Planning with reference to Simulink Clock for 3-second duration
    
    % Initial conditions (set to zero)
    q0 = 0;      % Initial Position
    qd0 = 0;     % Initial Velocity
    qdd0 = 0;    % Initial Acceleration
    qdf = 0;     % Final Velocity
    qddf = 0;    % Final Acceleration
    
    % Total time for trajectory
    T = 0.5;  % 3 seconds duration
    
    % Clamp time to ensure it does not exceed 3 seconds
    t = min(t, T);
    
    % Polynomial coefficients calculation based on boundary conditions
    a0 = q0;
    a1 = qd0;
    a2 = qdd0 / 2;
    a3 = (20 * qf - 20 * q0 - 8 * qdf - 12 * qd0 - 3 * qdd0 + qddf) / (2 * T^3);
    a4 = (30 * q0 - 30 * qf + 14 * qdf + 16 * qd0 + 3 * qdd0 - 2 * qddf) / (2 * T^4);
    a5 = (12 * qf - 12 * q0 - 6 * qdf - 6 * qd0 - qdd0 + qddf) / (2 * T^5);
    
    % Calculate position, velocity, and acceleration based on time t
    q = a0 + a1 * t + a2 * t^2 + a3 * t^3 + a4 * t^4 + a5 * t^5;
    qd = a1 + 2 * a2 * t + 3 * a3 * t^2 + 4 * a4 * t^3 + 5 * a5 * t^4;
    qdd = 2 * a2 + 6 * a3 * t + 12 * a4 * t^2 + 20 * a5 * t^3;
    
    % Ensure the final position q reaches qf exactly after 3 seconds
    if t == T
        q = qf;
        qd = 0;  % Final velocity is zero if not specified
        qdd = 0; % Final acceleration is zero if not specified
    end
end

== matlab function Test_simulation_model_backhoe/Trajectory/MATLAB Function3 ==
  data: qf input; q output; t input; qd output; qdd output
function [q, qd, qdd] = quintic_trajectory_planning(qf, t)
    % Quintic Trajectory Planning with reference to Simulink Clock for 3-second duration
    
    % Initial conditions (set to zero)
    q0 = 0;      % Initial Position
    qd0 = 0;     % Initial Velocity
    qdd0 = 0;    % Initial Acceleration
    qdf = 0;     % Final Velocity
    qddf = 0;    % Final Acceleration
    
    % Total time for trajectory
    T = 0.5;  % 3 seconds duration
    
    % Clamp time to ensure it does not exceed 3 seconds
    t = min(t, T);
    
    % Polynomial coefficients calculation based on boundary conditions
    a0 = q0;
    a1 = qd0;
    a2 = qdd0 / 2;
    a3 = (20 * qf - 20 * q0 - 8 * qdf - 12 * qd0 - 3 * qdd0 + qddf) / (2 * T^3);
    a4 = (30 * q0 - 30 * qf + 14 * qdf + 16 * qd0 + 3 * qdd0 - 2 * qddf) / (2 * T^4);
    a5 = (12 * qf - 12 * q0 - 6 * qdf - 6 * qd0 - qdd0 + qddf) / (2 * T^5);
    
    % Calculate position, velocity, and acceleration based on time t
    q = a0 + a1 * t + a2 * t^2 + a3 * t^3 + a4 * t^4 + a5 * t^5;
    qd = a1 + 2 * a2 * t + 3 * a3 * t^2 + 4 * a4 * t^3 + 5 * a5 * t^4;
    qdd = 2 * a2 + 6 * a3 * t + 12 * a4 * t^2 + 20 * a5 * t^3;
    
    % Ensure the final position q reaches qf exactly after 3 seconds
    if t == T
        q = qf;
        qd = 0;  % Final velocity is zero if not specified
        qdd = 0; % Final acceleration is zero if not specified
    end
end
